simulink model "acs6123_m5"  (Simulink 9.1)
settings: Solver=ode45  StartTime=0.0  StopTime=300  MaxStep=1  RelTol=1e-3  AbsTol=1e-3  EnableMultiTasking=on
settings Model: Creator=Brian  LastModifiedBy=Brian  ExtModeTrigMode=oneshot  ExtModeArmWhenConnect=off
settings SolverCC: AutoScaleAbsTol=off
settings DataIOCC: SignalLoggingSaveFormat=ModelDataLogs  SaveOutput=off  SaveTime=off  SignalLoggingName=sigsOut
settings OptimizationCC: BooleanDataType=off  LifeSpan=auto
settings DebuggingCC: SaveWithParameterizedLinksMsg=none  SignalResolutionControl=TryResolveAllWithWarning  MultiTaskDSMMsg=warning  MultiTaskCondExecSysMsg=none  SFUnexpectedBacktrackingDiag=error  SFNoUnconditionalDefaultTransitionDiag=error  SFExecutionAtInitializationDiag=warning
settings HardwareCC: TargetUnknown=on
settings CodeAppCC: StateflowObjectComments=off

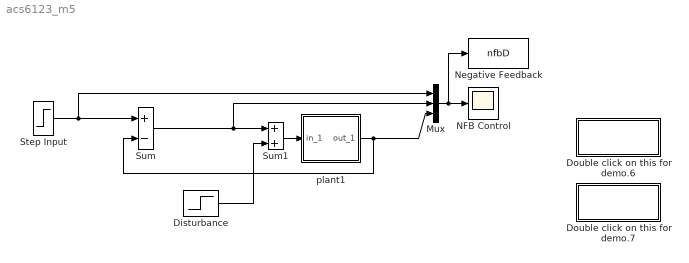
== system acs6123_m5 ==
  Disturbance : Step  Time=150  After=0  SampleTime=0
  Double click on this for demo.6 : Subsystem
      settings: OpenFcn=fuzzy patient
      mask Display: disp('Edit\n Fuzzy Rules')
  Double click on this for demo.7 : Subsystem
      settings: OpenFcn=readrls
      mask Display: disp('Compile\n Fuzzy Rules')
  Mux : Mux  Inputs=3
  NFB Control : Scope
  Negative Feedback : ToWorkspace  VariableName=nfbD  SaveFormat=Timeseries  SampleTime=-1
  Step Input : Step  Time=0  After=0.8  SampleTime=0
  Sum : Sum  Inputs=+-  SaturateOnIntegerOverflow=on  InputSameDT=on  OutDataTypeStr=Inherit: Same as first input
  Sum1 : Sum  SaturateOnIntegerOverflow=on  InputSameDT=on  OutDataTypeStr=Inherit: Same as first input
  plant1 : Subsystem
      mask Display: disp('Patient')
  wires:
  Step Input/1 -> Sum/1, Mux/1
  Sum1/1 -> plant1/1(in_1)
  Disturbance/1 -> Sum1/2
  Sum/1 -> Sum1/1, Mux/2
  Mux/1 -> Negative Feedback/1, NFB Control/1
  plant1/1(out_1) -> Sum/2, Mux/3

== system acs6123_m5/Double click on this for demo.6 ==

== system acs6123_m5/Double click on this for demo.7 ==

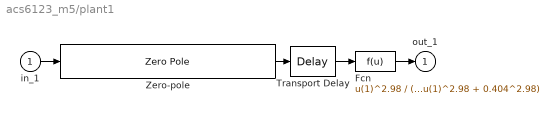
== system acs6123_m5/plant1 ==
  in_1 : Inport
  Fcn : Fcn  Expr=u(1)^2.98 / (u(1)^2.98 + 0.404^2.98)
  Transport Delay : TransportDelay
  Zero-pole : ZeroPole  Zeros=[-1/10.6]  Poles=[-1/34.42; -1/3.08; -1/4.81]  Gain=[10.64/(34.42*3.08*4.81)]
  out_1 : Outport
  wires:
  Zero-pole/1 -> Transport Delay/1
  Transport Delay/1 -> Fcn/1
  in_1/1 -> Zero-pole/1
  Fcn/1 -> out_1/1
